simulink model "simulink_Feedback_integral"  (R2023b)
settings: Solver=ode4  StartTime=0.0  StopTime=50  FixedStep=0.02  RelTol=1e-3
settings Model: Creator=PC  LastModifiedBy=q
settings SolverCC: AlgebraicLoopSolver=TrustRegion
settings DebuggingCC: UnconnectedInputMsg=warning  UnconnectedOutputMsg=warning  UnconnectedLineMsg=warning  ArithmeticOperatorsInVariantConditions=warning
settings ModelReferenceCC: EnableRefExpFcnMdlSchedulingChecks=on
settings SFSimCC: CustomCodeUndefinedFunction=UseInterfaceOnly
settings CodeAppCC: StateflowObjectComments=on

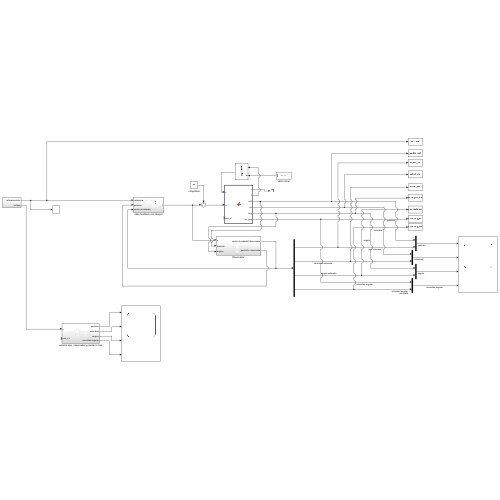
[thumbnail: Simulink's stored preview of the top-level diagram]
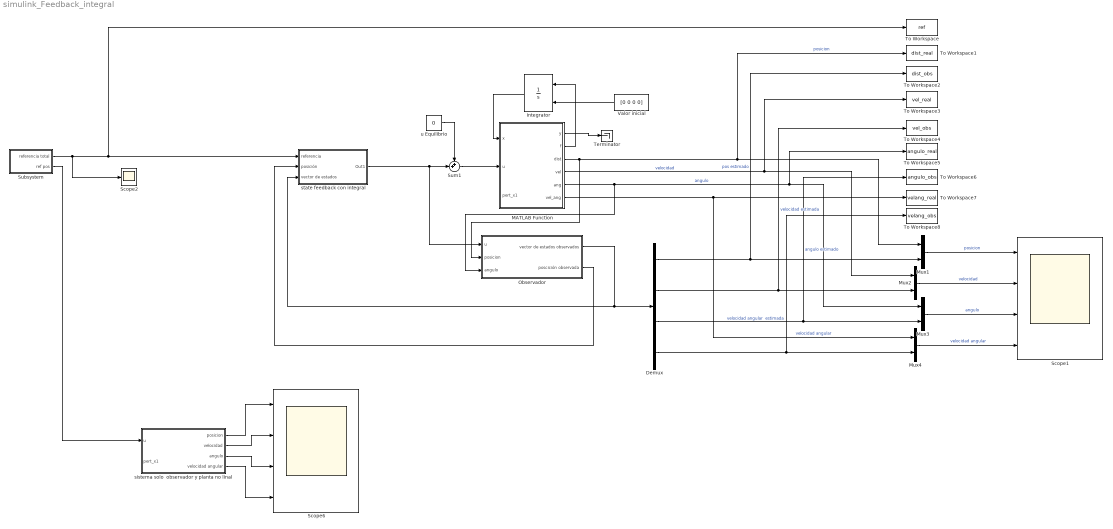
== system simulink_Feedback_integral ==
  Demux : Demux
  Integrator : Integrator  InitialConditionSource=external
  MATLAB Function : MATLAB Function  TreatAsAtomicUnit=on
  Mux{1..4} (4 alike) : Mux  Inputs=2
  "Observador " : Subsystem
  Scope1 : Scope  NumInputPorts=4
  Scope2 : Scope
  Scope6 : Scope  NumInputPorts=4
  Subsystem : Subsystem
  Sum1 : Sum  Inputs=++|
  Terminator : Terminator
  To Workspace : ToWorkspace  VariableName=ref  SampleTime=0.02
  To Workspace1 : ToWorkspace  VariableName=dist_real  SampleTime=0.02
  To Workspace2 : ToWorkspace  VariableName=dist_obs  SampleTime=0.02
  To Workspace3 : ToWorkspace  VariableName=vel_real  SampleTime=0.02
  To Workspace4 : ToWorkspace  VariableName=vel_obs  SampleTime=0.02
  To Workspace5 : ToWorkspace  VariableName=angulo_real  SampleTime=0.02
  To Workspace6 : ToWorkspace  VariableName=angulo_obs  SampleTime=0.02
  To Workspace7 : ToWorkspace  VariableName=velang_real  SampleTime=0.02
  To Workspace8 : ToWorkspace  VariableName=velang_obs  SampleTime=0.02
  Valor inicial : Constant  Value=[0 0 0 0]
  sistema solo  observador y planta no linal : Subsystem
  state feedback con integral : Subsystem
  u Equilibrio : Constant  Value=0
  wires:
  Valor inicial/1 -> Integrator/2
  MATLAB Function/2(f) -> Integrator/1
  u Equilibrio/1 -> Sum1/1
  Sum1/1 -> MATLAB Function/2(u)
  Integrator/1 -> MATLAB Function/1(x)
  MATLAB Function/6(vel_ang) -> To Workspace7/1, Mux4/1  "velocidad angular"
  Demux/4 -> To Workspace8/1, Mux4/2  "velocidad angular  estimada"
  Mux1/1 -> Scope1/1  "posicion"
  Demux/1 -> Mux1/2, To Workspace2/1  "pos estimado"
  Mux2/1 -> Scope1/2  "velocidad"
  Mux4/1 -> Scope1/4  "velocidad angular"
  Demux/2 -> Mux2/2, To Workspace4/1  "velocidad estimada"
  Demux/3 -> To Workspace6/1, Mux3/2  "angulo estimado"
  MATLAB Function/5(ang) -> To Workspace5/1, Mux3/1, "Observador "/3(angulo)  "angulo"
  Mux3/1 -> Scope1/3  "angulo"
  MATLAB Function/4(vel) -> To Workspace3/1, Mux2/1  "velocidad"
  MATLAB Function/3(dist) -> "Observador "/2(posicion), To Workspace1/1, Mux1/1  "posicion"
  MATLAB Function/1(y) -> Terminator/1
  "Observador "/1(vector de estados observados) -> state feedback con integral/3(vector de estados), Demux/1
  sistema solo  observador y planta no linal/1(posicion) -> Scope6/1
  sistema solo  observador y planta no linal/2(velocidad) -> Scope6/2
  sistema solo  observador y planta no linal/3(angulo) -> Scope6/3
  sistema solo  observador y planta no linal/4(velocidad angular) -> Scope6/4
  state feedback con integral/1(Out1) -> "Observador "/1(u), Sum1/2
  "Observador "/2(poscición observada) -> state feedback con integral/2(posición)
  Subsystem/1(referencia total) -> Scope2/1, state feedback con integral/1(referencia), To Workspace/1
  Subsystem/2(ref pos) -> sistema solo  observador y planta no linal/1(u)

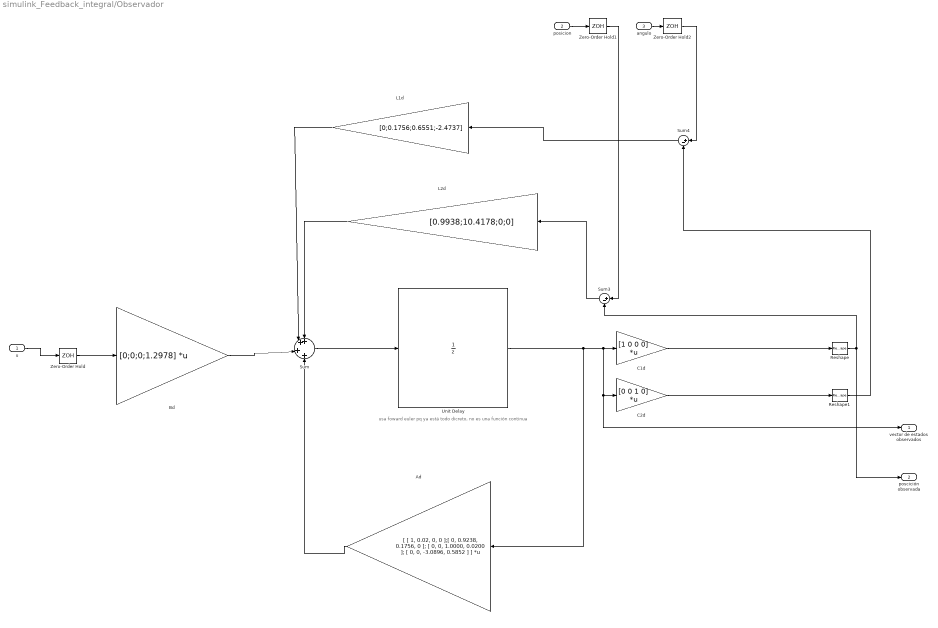
== system simulink_Feedback_integral/Observador  ==
  note: usa foward euler pq ya está todo dicreto, no es una función continua
  u : Inport
  posicion : Inport  Port=2
  angulo : Inport  Port=3
  Ad : Gain  Gain=|  Multiplication=Matrix(K*u)
      | [ [ 1, 0.02, 0, 0 ];[ 0, 0.9238, 0.1756, 0 ];
      | [ 0, 0, 1.0000, 0.0200 ]; [ 0, 0, -3.0896, 0.5852 ] ]
  Bd : Gain  Gain=[0;0;0;1.2978]  Multiplication=Matrix(K*u)
  C1d : Gain  Gain=[1 0 0 0]  Multiplication=Matrix(K*u)
  C2d : Gain  Gain=[0 0 1 0]  Multiplication=Matrix(K*u)
  L1d : Gain  Gain=[0;0.1756;0.6551;-2.4737]
  L2d : Gain  Gain=[0.9938;10.4178;0;0]
  Reshape : Reshape
  Reshape1 : Reshape  OutputDimensions=[1]
  Sum : Sum  Inputs=++|+|+
  Sum3 : Sum  Inputs=|+-
  Sum4 : Sum  Inputs=|+-
  Unit Delay : UnitDelay  SampleTime=0.02  HasFrameUpgradeWarning=on
  Zero-Order Hold : ZeroOrderHold  SampleTime=0.02
  Zero-Order Hold1 : ZeroOrderHold  SampleTime=0.02
  Zero-Order Hold2 : ZeroOrderHold  SampleTime=0.02
  vector de estados observados : Outport  VectorParamsAs1DForOutWhenUnconnected=off
  poscición observada : Outport  Port=2  VectorParamsAs1DForOutWhenUnconnected=off
  wires:
  Ad/1 -> Sum/4
  Sum/1 -> Unit Delay/1
  Bd/1 -> Sum/3
  Unit Delay/1 -> C2d/1, vector de estados observados/1, C1d/1, Ad/1
  Sum4/1 -> L1d/1
  L2d/1 -> Sum/1
  C2d/1 -> Reshape1/1
  Reshape/1 -> poscición observada/1, Sum3/2
  Sum3/1 -> L2d/1
  L1d/1 -> Sum/2
  Reshape1/1 -> Sum4/2
  C1d/1 -> Reshape/1
  angulo/1 -> Zero-Order Hold2/1
  posicion/1 -> Zero-Order Hold1/1
  u/1 -> Zero-Order Hold/1
  Zero-Order Hold/1 -> Bd/1
  Zero-Order Hold1/1 -> Sum3/1
  Zero-Order Hold2/1 -> Sum4/1

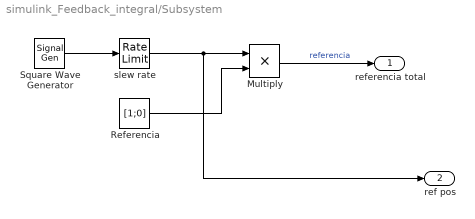
== system simulink_Feedback_integral/Subsystem ==
  Multiply : Product
  Referencia : Constant  Value=[1;0]
  Square Wave Generator : SignalGenerator  WaveForm=square  Amplitude=-0.08  Frequency=0.125
  slew rate : RateLimiter  RisingSlewLimit=0.1  FallingSlewLimit=-0.1  SampleTimeMode=inherited
  referencia total : Outport
  ref pos : Outport  Port=2
  wires:
  Square Wave Generator/1 -> slew rate/1
  slew rate/1 -> ref pos/1, Multiply/1
  Multiply/1 -> referencia total/1  "referencia"
  Referencia/1 -> Multiply/2

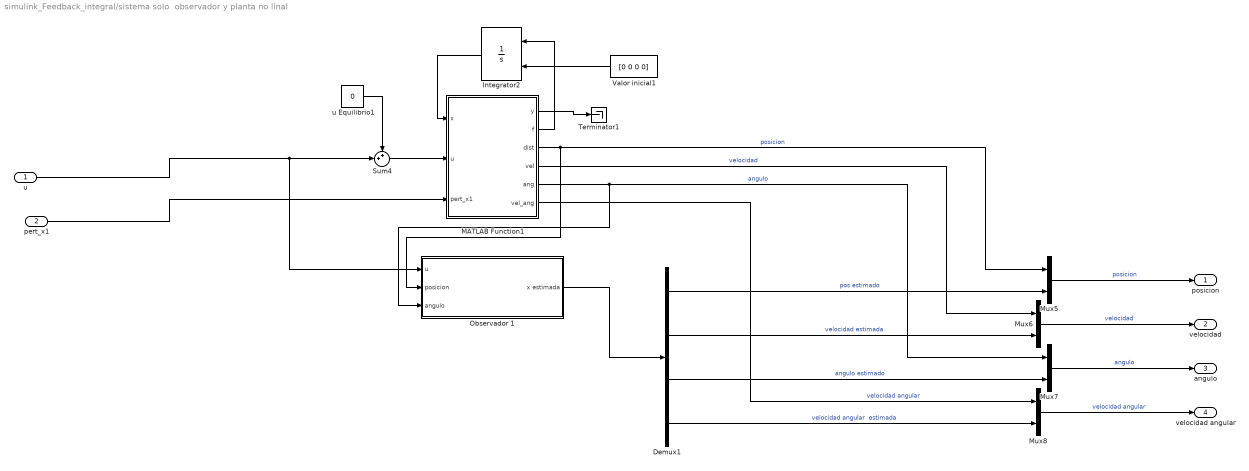
== system simulink_Feedback_integral/sistema solo  observador y planta no linal ==
  u : Inport
  pert_x1 : Inport  Port=2
  Demux1 : Demux
  Integrator2 : Integrator  InitialConditionSource=external
  MATLAB Function1 : MATLAB Function  TreatAsAtomicUnit=on
  Mux{5..8} (4 alike) : Mux  Inputs=2
  Observador 1 : Subsystem
  Sum4 : Sum  Inputs=++|
  Terminator1 : Terminator
  Valor inicial1 : Constant  Value=[0 0 0 0]
  u Equilibrio1 : Constant  Value=0
  posicion : Outport
  velocidad : Outport  Port=2
  angulo : Outport  Port=3
  velocidad angular : Outport  Port=4
  wires:
  Integrator2/1 -> MATLAB Function1/1(x)
  Observador 1/1(x estimada) -> Demux1/1
  Mux5/1 -> posicion/1  "posicion"
  u Equilibrio1/1 -> Sum4/1
  Sum4/1 -> MATLAB Function1/2(u)
  MATLAB Function1/4(vel) -> Mux6/1  "velocidad"
  MATLAB Function1/3(dist) -> Mux5/1, Observador 1/2(posicion)  "posicion"
  MATLAB Function1/1(y) -> Terminator1/1
  MATLAB Function1/6(vel_ang) -> Mux8/1  "velocidad angular"
  Demux1/4 -> Mux8/2  "velocidad angular  estimada"
  Valor inicial1/1 -> Integrator2/2
  MATLAB Function1/2(f) -> Integrator2/1
  Demux1/3 -> Mux7/2  "angulo estimado"
  MATLAB Function1/5(ang) -> Observador 1/3(angulo), Mux7/1  "angulo"
  Mux7/1 -> angulo/1  "angulo"
  Demux1/2 -> Mux6/2  "velocidad estimada"
  Demux1/1 -> Mux5/2  "pos estimado"
  Mux6/1 -> velocidad/1  "velocidad"
  u/1 -> Observador 1/1(u), Sum4/2
  Mux8/1 -> velocidad angular/1  "velocidad angular"
  pert_x1/1 -> MATLAB Function1/3(pert_x1)

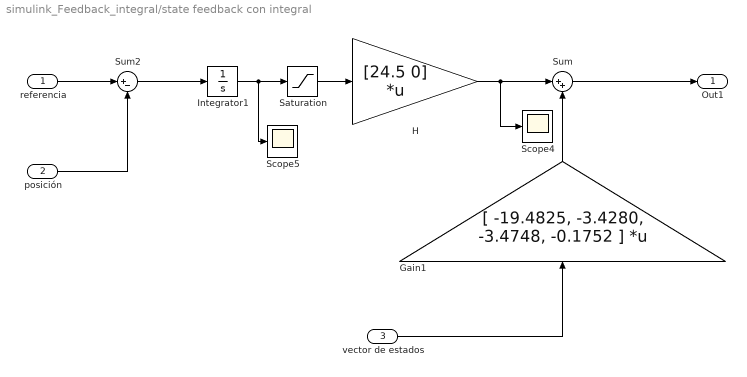
== system simulink_Feedback_integral/state feedback con integral ==
  referencia : Inport
  posición : Inport  Port=2
  vector de estados : Inport  Port=3
  Gain1 : Gain  Gain=[ -19.4825, -3.4280, -3.4748, -0.1752 ]  Multiplication=Matrix(K*u)
  H : Gain  Gain=[24.5 0]  Multiplication=Matrix(K*u)
  Integrator1 : Integrator
  Saturation : Saturate  UpperLimit=2.4  LowerLimit=-2.4
  Scope4 : Scope
  Scope5 : Scope
  Sum : Sum  Inputs=|++
  Sum2 : Sum  Inputs=|+-
  Out1 : Outport
  wires:
  Integrator1/1 -> Scope5/1, Saturation/1
  Saturation/1 -> H/1
  Gain1/1 -> Sum/2
  Sum2/1 -> Integrator1/1
  referencia/1 -> Sum2/1
  posición/1 -> Sum2/2
  H/1 -> Sum/1, Scope4/1
  Sum/1 -> Out1/1
  vector de estados/1 -> Gain1/1

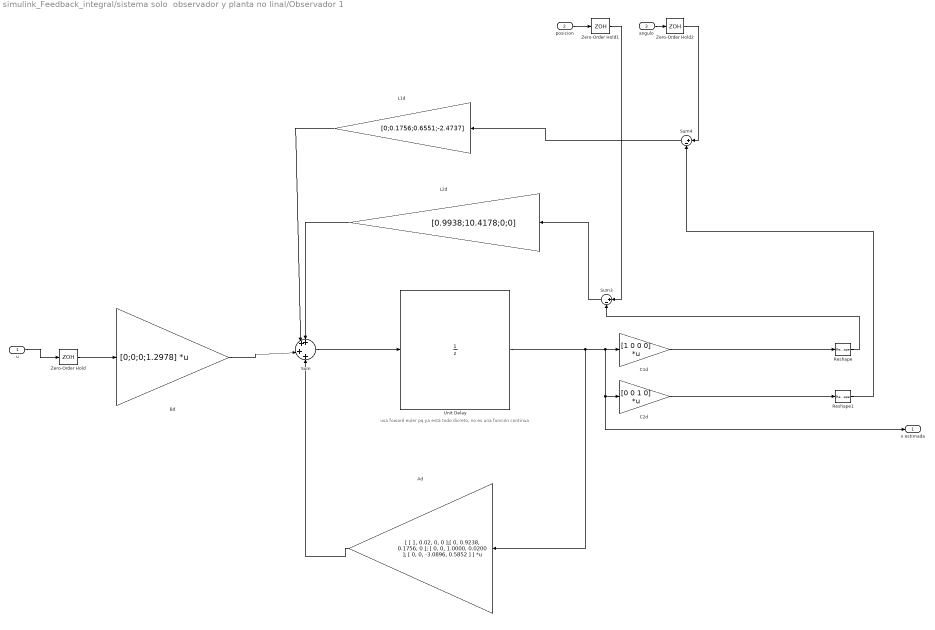
== system simulink_Feedback_integral/sistema solo  observador y planta no linal/Observador 1 ==
  note: usa foward euler pq ya está todo dicreto, no es una función continua
  u : Inport
  posicion : Inport  Port=2
  angulo : Inport  Port=3
  Ad : Gain  Gain=|  Multiplication=Matrix(K*u)
      | [ [ 1, 0.02, 0, 0 ];[ 0, 0.9238, 0.1756, 0 ];
      | [ 0, 0, 1.0000, 0.0200 ]; [ 0, 0, -3.0896, 0.5852 ] ]
  Bd : Gain  Gain=[0;0;0;1.2978]  Multiplication=Matrix(K*u)
  C1d : Gain  Gain=[1 0 0 0]  Multiplication=Matrix(K*u)
  C2d : Gain  Gain=[0 0 1 0]  Multiplication=Matrix(K*u)
  L1d : Gain  Gain=[0;0.1756;0.6551;-2.4737]
  L2d : Gain  Gain=[0.9938;10.4178;0;0]
  Reshape : Reshape
  Reshape1 : Reshape  OutputDimensions=[1]
  Sum : Sum  Inputs=++|+|+
  Sum3 : Sum  Inputs=|+-
  Sum4 : Sum  Inputs=|+-
  Unit Delay : UnitDelay  SampleTime=0.02  HasFrameUpgradeWarning=on
  Zero-Order Hold : ZeroOrderHold  SampleTime=0.02
  Zero-Order Hold1 : ZeroOrderHold  SampleTime=0.02
  Zero-Order Hold2 : ZeroOrderHold  SampleTime=0.02
  x estimada : Outport  VectorParamsAs1DForOutWhenUnconnected=off
  wires:
  Zero-Order Hold2/1 -> Sum4/1
  Zero-Order Hold1/1 -> Sum3/1
  Zero-Order Hold/1 -> Bd/1
  u/1 -> Zero-Order Hold/1
  posicion/1 -> Zero-Order Hold1/1
  angulo/1 -> Zero-Order Hold2/1
  C1d/1 -> Reshape/1
  Reshape1/1 -> Sum4/2
  L1d/1 -> Sum/2
  Sum3/1 -> L2d/1
  Reshape/1 -> Sum3/2
  C2d/1 -> Reshape1/1
  L2d/1 -> Sum/1
  Sum4/1 -> L1d/1
  Unit Delay/1 -> Ad/1, C1d/1, x estimada/1, C2d/1
  Bd/1 -> Sum/3
  Sum/1 -> Unit Delay/1
  Ad/1 -> Sum/4

== matlab function simulink_Feedback_integral/sistema solo  observador y planta no linal/MATLAB Function1 ==
  data: x input; u input; y output; f output; pert_x1 input; dist output; vel output; ang output; vel_ang output
function [y, f,dist,vel,ang,vel_ang] = fcn(x, u, pert_x1)
    
    g = 9.81; %kg m/s2
    m = 0.047; %kg
    kv = 0.2;
    R = 0.02;
    mr = 0.00275;
    J = 0.5*4*mr*power(R,2);
    
    x(1) = x(1) + pert_x1;

    %Dinamica
    f1 = x(2);
    f2 = (m*g*sin(x(3)) - kv * x(2)) * 1/(m + (J/power(R,2)));
    f3 = x(4);
    f4 = -20.73 * x(4) - 154.47*x(3) + u * 64.89;

    y = x(1);
    f = [f1 f2 f3 f4];
    dist=x(1);
    vel=x(2);
    ang=x(3);
    vel_ang=x(4);
end

== matlab function simulink_Feedback_integral/MATLAB Function ==
  data: x input; u input; y output; f output; pert_x1 input; dist output; vel output; ang output; vel_ang output
function [y, f,dist,vel,ang,vel_ang] = fcn(x, u, pert_x1)
    
    g = 9.81; %kg m/s2
    m = 0.047; %kg
    kv = 0.2;
    R = 0.02;
    mr = 0.00275;
    J = 0.5*4*mr*power(R,2);
    
    x(1) = x(1) + pert_x1;

    %Dinamica
    f1 = x(2);
    f2 = (m*g*sin(x(3)) - kv * x(2)) * 1/(m + (J/power(R,2)));
    f3 = x(4);
    f4 = -20.73 * x(4) - 154.47*x(3) + u * 64.89;

    y = x(1);
    f = [f1 f2 f3 f4];
    dist=x(1);
    vel=x(2);
    ang=x(3);
    vel_ang=x(4);
end
